simulink model "three_phase_dab"  (R2025b)
settings: Solver=ode23tb  StartTime=0.0  StopTime=simlength  FixedStep=tc  MaxStep=tc
values from neighbouring files (symbols this model uses):
  Idc_FS = max(Idab1_dc_nom,Idab2_dc_nom) * margin_factor    [init_model.m]
  tc = ts_dab/100    (= 4.16666666667e-07)    [init_model.m]
  Vdab2_dc_nom = 1500    [init_model.m]
  Vdc_FS = max(Vdab1_dc_nom,Vdab2_dc_nom) * margin_factor    [init_model.m]
libraries: fl_lib x19, nesl_utility x15, discrete_time_low_pass_filter x6, single_phase_transformer_lib x3, litium_ion_battery x2, pi_ctrl x2, three_phase_inverter_ideal_switch_based_model x2, three_phase_inverter_mosfet_based_with_thermal_model x2, three_phase_dab_modulator x1
settings Model: SimulationMode=accelerator  Creator=LTNBDA  LastModifiedBy=ltnbda
settings SolverCC: ZeroCrossControl=EnableAll  ZeroCrossAlgorithm=Adaptive  AlgebraicLoopSolver=TrustRegion  SolverResetMethod=Robust  AutoInsertRateTranBlk=on
settings DataIOCC: LimitDataPoints=on  MaxDataPoints=1  SaveFormat=Array  SignalLoggingSaveFormat=ModelDataLogs  SaveOutput=off  SignalLogging=off  DSMLogging=off  SaveTime=off  ReturnWorkspaceOutputs=off
settings OptimizationCC: ExpressionDepthLimit=2147483647.0  InitFltsAndDblsToZero=on  EfficientMapNaN2IntZero=off  LifeSpan=inf
settings DebuggingCC: SaveWithParameterizedLinksMsg=none  UnderspecifiedInitializationDetection=Classic  MergeDetectMultiDrivingBlocksExec=none  SignalResolutionControl=TryResolveAllWithWarning  SolverPrmCheckMsg=warning  MultiTaskDSMMsg=warning  MultiTaskCondExecSysMsg=none  MultiTaskRateTransMsg=warning  FcnCallInpInsideContextMsg=warning  StateNameClashWarn=warning  SFUnexpectedBacktrackingDiag=warning  SFNoUnconditionalDefaultTransitionDiag=warning  ArithmeticOperatorsInVariantConditions=warning
settings HardwareCC: ProdBitPerLong=64.0  ProdLargestAtomicFloat=None  ProdIntDivRoundTo=Undefined  ProdEndianess=Unspecified  ProdHWDeviceType=Generic->64-bit Embedded Processor (LP64)  TargetBitPerPointer=64.0  TargetBitPerSizeT=64.0  TargetBitPerPtrDiffT=64.0  TargetLongLongMode=on  TargetIntDivRoundTo=Zero  TargetEndianess=LittleEndian  TargetWordSize=64.0  TargetHWDeviceType=MATLAB Host  ProdEqTarget=off
settings ModelReferenceCC: EnableRefExpFcnMdlSchedulingChecks=on  PropagateSignalLabelsOutOfModel=off
settings SFSimCC: SimUseLocalCustomCode=off  CustomCodeUndefinedFunction=UseInterfaceOnly
settings RTWCC: RTWUseLocalCustomCode=off  GPUComputeCapability=3.5
settings CodeAppCC: MaxIdLength=128.0  StateflowObjectComments=on
settings GRTTargetCC: TargetLangStandard=C89/C90 (ANSI)  CombineOutputUpdateFcns=off  GRTInterface=on
settings ConfigComp: CovMetricSettings=dw  CovSaveCumulativeToWorkspaceVar=on  CovSaveSingleToWorkspaceVar=on  CovExternalEMLEnable=off
settings SimscapeCC: SimscapeNormalizeSystem=off

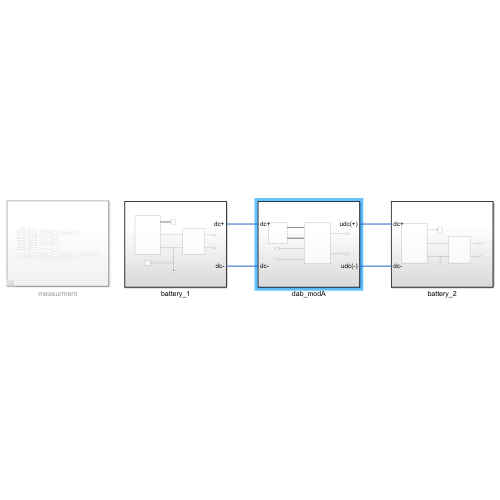
[thumbnail: Simulink's stored preview of the top-level diagram]
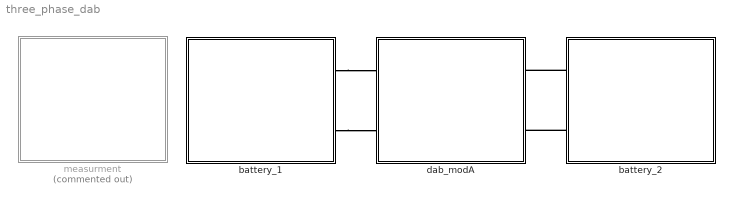
== system three_phase_dab ==
  battery_1 : Subsystem
  battery_2 : Subsystem
  dab_modA : Subsystem
  measurment : Subsystem  Commented=on
  connections:
  battery_2/RConn2 -- dab_modA/RConn2
  battery_2/RConn1 -- dab_modA/RConn1
  battery_1/RConn1 -- dab_modA/LConn1
  battery_1/RConn2 -- dab_modA/LConn2

== system three_phase_dab/battery_1 ==
  Electrical Reference1 : fl_lib/Electrical/Electrical Elements/Electrical Reference
  Solver Configuration : nesl_utility/Solver Configuration  PhysicalDomain=network_engine_domain  SubClassName=solver  LeftPortType=input  RightPortType=generic  Tones=[]  Harmonics=[]  SimulateNoise=off  Profile=off  UseLocalSampling=off  EnableSwitchedLinearOptims=on  FrequencyDomain=off  UseCCode=off  RelTol=0.001  AbsTol=0.001  MinStep=1e-09  ToWorkspace=off  RevertToSquareIcSolve=off  NumHomotopyIterations=100  PhasorMode=off  PhasorModeNumHarmonics=1  ConsistencySolver=NEWTON_FTOL  IndexReductionMethod=DerivativeReplacement  DoDC=off  ResidualTolerance=1e-09  ConsistencyTolSource=GLOBAL  ConsistencyAbsTol=0.001  ConsistencyRelTol=0.001  ConsistencyTolFactor=0.001  UseLocalSolver=on  LocalSolverChoice=NE_BACKWARD_EULER_ADVANCER  ResolveIndetEquations=on  FunctionEvalNumThread=1  LocalSolverSampleTime=tc  DoFixedCost=on  MaxNonlinIter=3  MaxModeIter=2  ComputeImpulses=off  ImpulseIterations=2  LinearAlgebra=auto  LinearAlgebraNumThread=0  EquationFormulation=NE_TIME_EF  DelaysMemoryBudget=1024  AutomaticFiltering=on  FilteringTimeConstant=0.001  PartitionStorageMethod=AS_NEEDED  PartitionMemoryBudget=1024  PartitionMethod=ROBUST  MultibodyUseLocalSolver=off  MultibodyLocalSolverChoice=ODE1  MultibodyLocalSolverSampleTime=0.001
  litium ion battery 1 : Scope
      settings: ActiveDisplayYMinimum=1095.5241232297076  ActiveDisplayYMaximum=1432.6160946881369  DataLoggingVariableName=ScopeData3
  litium_ion_battery : litium_ion_battery/litium_ion_battery  Q=50  number_of_cells=346  E_1=-1.031  E0=3.485  E1=0  E2=0  E3=0  Elog=-0.05  R0=0.035  R1=0.035  C1=0.5  M=125  alpha=35  soc_init=0.85  ts_battery=ts_battery  q1Kalman=q1Kalman  q2Kalman=q2Kalman  q3Kalman=q3Kalman  rKalman=rKalman  tc=tc
  single_phase_ui_measure : Subsystem
  dc+ : PMIOPort  Side=Right
  dc- : PMIOPort  Port=2  Side=Right
  wires:
  litium_ion_battery/1 -> litium ion battery 1/1
  connections:
  litium_ion_battery/RConn2 -- single_phase_ui_measure/LConn2 -- Electrical Reference1/LConn1 -- Solver Configuration/RConn1
  single_phase_ui_measure/RConn1 -- dc+/RConn1
  single_phase_ui_measure/LConn1 -- litium_ion_battery/RConn1
  dc-/RConn1 -- single_phase_ui_measure/RConn2

== system three_phase_dab/battery_2 ==
  Electrical Reference1 : fl_lib/Electrical/Electrical Elements/Electrical Reference
  litium ion battery 2 : Scope
      settings: ActiveDisplayYMinimum=-748.38980710578858  ActiveDisplayYMaximum=3166.4304287109808  DataLoggingVariableName=ScopeData3
  litium_ion_battery : litium_ion_battery/litium_ion_battery  Q=50  number_of_cells=346  E_1=-1.031  E0=3.485  E1=0  E2=0  E3=0  Elog=-0.05  R0=0.035  R1=0.035  C1=0.5  M=125  alpha=35  soc_init=0.85  ts_battery=ts_battery  q1Kalman=q1Kalman  q2Kalman=q2Kalman  q3Kalman=q3Kalman  rKalman=rKalman  tc=tc
  single_phase_ui_measure : Subsystem
  dc+ : PMIOPort  Side=Right
  dc- : PMIOPort  Port=2  Side=Right
  wires:
  litium_ion_battery/1 -> litium ion battery 2/1
  connections:
  dc-/RConn1 -- single_phase_ui_measure/RConn2
  single_phase_ui_measure/LConn1 -- litium_ion_battery/RConn1
  single_phase_ui_measure/RConn1 -- dc+/RConn1
  Electrical Reference1/LConn1 -- single_phase_ui_measure/LConn2 -- litium_ion_battery/RConn2

== system three_phase_dab/dab_modA ==
  dab_ctrl : Subsystem
  dcdc_with_galvanic_isolation : Subsystem
  udc(+) : PMIOPort  Side=Right
  udc(-) : PMIOPort  Port=2  Side=Right
  dc+ : PMIOPort  Port=3  Side=Left
  dc- : PMIOPort  Port=4  Side=Left
  wires:
  dab_ctrl/2(gate_commands_2) -> dcdc_with_galvanic_isolation/2(gate_commands_1)
  dab_ctrl/1(gate_commands_1) -> dcdc_with_galvanic_isolation/1(gate_commands_2)
  connections:
  udc(+)/RConn1 -- dcdc_with_galvanic_isolation/RConn1
  udc(-)/RConn1 -- dcdc_with_galvanic_isolation/RConn2
  dc-/RConn1 -- dcdc_with_galvanic_isolation/LConn2
  dc+/RConn1 -- dcdc_with_galvanic_isolation/LConn1

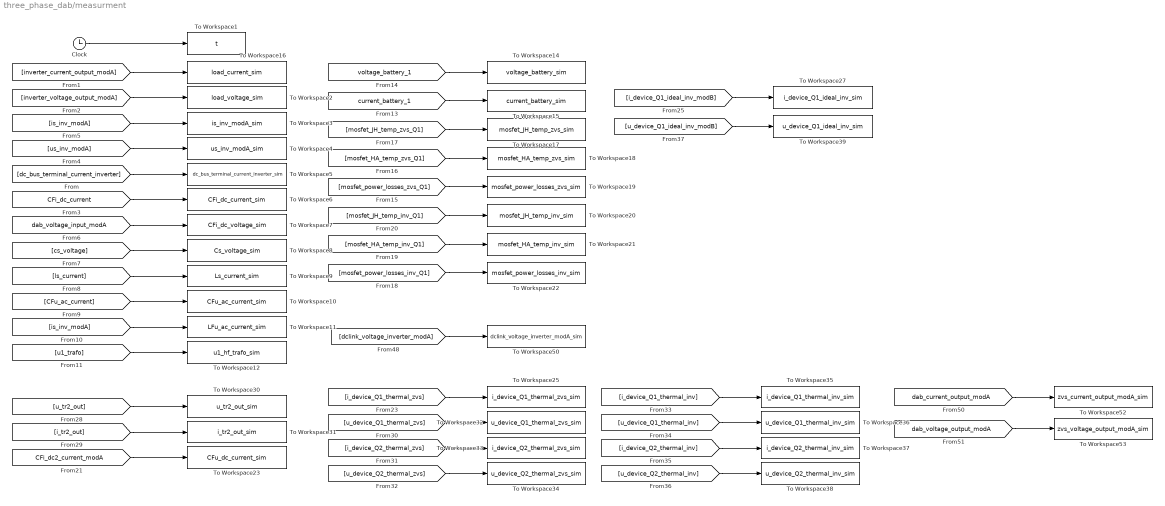
== system three_phase_dab/measurment ==
  Clock : Clock
  To Workspace1 : ToWorkspace  VariableName=t  SampleTime=tc
      settings: MaxDataPoints=Nc
  To Workspace10 : ToWorkspace  VariableName=CFu_ac_current_sim  SampleTime=tc
      settings: MaxDataPoints=Nc
  To Workspace11 : ToWorkspace  VariableName=LFu_ac_current_sim  SampleTime=tc
      settings: MaxDataPoints=Nc
  To Workspace12 : ToWorkspace  VariableName=u1_hf_trafo_sim  SampleTime=tc
      settings: MaxDataPoints=Nc
  To Workspace14 : ToWorkspace  VariableName=voltage_battery_sim  SampleTime=tc
      settings: MaxDataPoints=Nc
  To Workspace15 : ToWorkspace  VariableName=current_battery_sim  SampleTime=tc
      settings: MaxDataPoints=Nc
  To Workspace16 : ToWorkspace  VariableName=load_current_sim  SampleTime=tc
      settings: MaxDataPoints=Nc
  To Workspace17 : ToWorkspace  VariableName=mosfet_JH_temp_zvs_sim  SampleTime=tc
      settings: MaxDataPoints=Nc
  To Workspace18 : ToWorkspace  VariableName=mosfet_HA_temp_zvs_sim  SampleTime=tc
      settings: MaxDataPoints=Nc
  To Workspace19 : ToWorkspace  VariableName=mosfet_power_losses_zvs_sim  SampleTime=tc
      settings: MaxDataPoints=Nc
  To Workspace2 : ToWorkspace  VariableName=load_voltage_sim  SampleTime=tc
      settings: MaxDataPoints=Nc
  To Workspace20 : ToWorkspace  VariableName=mosfet_JH_temp_inv_sim  SampleTime=tc
      settings: MaxDataPoints=Nc
  To Workspace21 : ToWorkspace  VariableName=mosfet_HA_temp_inv_sim  SampleTime=tc
      settings: MaxDataPoints=Nc
  To Workspace22 : ToWorkspace  VariableName=mosfet_power_losses_inv_sim  SampleTime=tc
      settings: MaxDataPoints=Nc
  To Workspace23 : ToWorkspace  VariableName=CFu_dc_current_sim  SampleTime=tc
      settings: MaxDataPoints=Nc
  To Workspace25 : ToWorkspace  VariableName=i_device_Q1_thermal_zvs_sim  SampleTime=tc
      settings: MaxDataPoints=Nc
  To Workspace27 : ToWorkspace  VariableName=i_device_Q1_ideal_inv_sim  SampleTime=tc
      settings: MaxDataPoints=Nc
  To Workspace3 : ToWorkspace  VariableName=is_inv_modA_sim  SampleTime=tc
      settings: MaxDataPoints=Nc
  To Workspace30 : ToWorkspace  VariableName=u_tr2_out_sim  SampleTime=tc
      settings: MaxDataPoints=Nc
  To Workspace31 : ToWorkspace  VariableName=i_tr2_out_sim  SampleTime=tc
      settings: MaxDataPoints=Nc
  To Workspace32 : ToWorkspace  VariableName=u_device_Q1_thermal_zvs_sim  SampleTime=tc
      settings: MaxDataPoints=Nc
  To Workspace33 : ToWorkspace  VariableName=i_device_Q2_thermal_zvs_sim  SampleTime=tc
      settings: MaxDataPoints=Nc
  To Workspace34 : ToWorkspace  VariableName=u_device_Q2_thermal_zvs_sim  SampleTime=tc
      settings: MaxDataPoints=Nc
  To Workspace35 : ToWorkspace  VariableName=i_device_Q1_thermal_inv_sim  SampleTime=tc
      settings: MaxDataPoints=Nc
  To Workspace36 : ToWorkspace  VariableName=u_device_Q1_thermal_inv_sim  SampleTime=tc
      settings: MaxDataPoints=Nc
  To Workspace37 : ToWorkspace  VariableName=i_device_Q2_thermal_inv_sim  SampleTime=tc
      settings: MaxDataPoints=Nc
  To Workspace38 : ToWorkspace  VariableName=u_device_Q2_thermal_inv_sim  SampleTime=tc
      settings: MaxDataPoints=Nc
  To Workspace39 : ToWorkspace  VariableName=u_device_Q1_ideal_inv_sim  SampleTime=tc
      settings: MaxDataPoints=Nc
  To Workspace4 : ToWorkspace  VariableName=us_inv_modA_sim  SampleTime=tc
      settings: MaxDataPoints=Nc
  To Workspace5 : ToWorkspace  VariableName=dc_bus_terminal_current_inverter_sim  SampleTime=tc
      settings: MaxDataPoints=Nc
  To Workspace50 : ToWorkspace  VariableName=dclink_voltage_inverter_modA_sim  SampleTime=tc
      settings: MaxDataPoints=Nc
  To Workspace52 : ToWorkspace  VariableName=zvs_current_output_modA_sim  SampleTime=tc
      settings: MaxDataPoints=Nc
  To Workspace53 : ToWorkspace  VariableName=zvs_voltage_output_modA_sim  SampleTime=tc
      settings: MaxDataPoints=Nc
  To Workspace6 : ToWorkspace  VariableName=CFi_dc_current_sim  SampleTime=tc
      settings: MaxDataPoints=Nc
  To Workspace7 : ToWorkspace  VariableName=CFi_dc_voltage_sim  SampleTime=tc
      settings: MaxDataPoints=Nc
  To Workspace8 : ToWorkspace  VariableName=Cs_voltage_sim  SampleTime=tc
      settings: MaxDataPoints=Nc
  To Workspace9 : ToWorkspace  VariableName=Ls_current_sim  SampleTime=tc
      settings: MaxDataPoints=Nc
  wires:
  Clock/1 -> To Workspace1/1
  [inverter_current_output_modA] -> To Workspace16/1
  [inverter_voltage_output_modA] -> To Workspace2/1
  [is_inv_modA] -> To Workspace3/1
  [us_inv_modA] -> To Workspace4/1
  [dc_bus_terminal_current_inverter] -> To Workspace5/1
  [CFi_dc_current] -> To Workspace6/1
  [dab_voltage_input_modA] -> To Workspace7/1
  [cs_voltage] -> To Workspace8/1
  [ls_current] -> To Workspace9/1
  [CFu_ac_current] -> To Workspace10/1
  [is_inv_modA] -> To Workspace11/1
  [u1_trafo] -> To Workspace12/1
  [voltage_battery_1] -> To Workspace14/1
  [current_battery_1] -> To Workspace15/1
  [mosfet_JH_temp_zvs_Q1] -> To Workspace17/1
  [mosfet_HA_temp_zvs_Q1] -> To Workspace18/1
  [mosfet_power_losses_zvs_Q1] -> To Workspace19/1
  [mosfet_power_losses_inv_Q1] -> To Workspace22/1
  [mosfet_HA_temp_inv_Q1] -> To Workspace21/1
  [mosfet_JH_temp_inv_Q1] -> To Workspace20/1
  [CFi_dc2_current_modA] -> To Workspace23/1
  [i_device_Q1_thermal_zvs] -> To Workspace25/1
  [i_device_Q1_ideal_inv_modB] -> To Workspace27/1
  [u_tr2_out] -> To Workspace30/1
  [i_tr2_out] -> To Workspace31/1
  [u_device_Q1_thermal_zvs] -> To Workspace32/1
  [u_device_Q2_thermal_zvs] -> To Workspace34/1
  [i_device_Q2_thermal_zvs] -> To Workspace33/1
  [i_device_Q2_thermal_inv] -> To Workspace37/1
  [u_device_Q2_thermal_inv] -> To Workspace38/1
  [u_device_Q1_thermal_inv] -> To Workspace36/1
  [i_device_Q1_thermal_inv] -> To Workspace35/1
  [u_device_Q1_ideal_inv_modB] -> To Workspace39/1
  [dclink_voltage_inverter_modA] -> To Workspace50/1
  [dab_voltage_output_modA] -> To Workspace53/1
  [dab_current_output_modA] -> To Workspace52/1

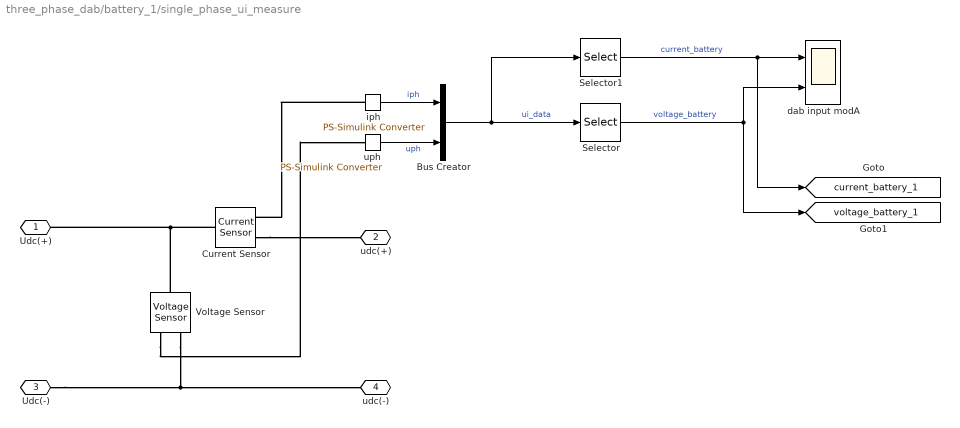
== system three_phase_dab/battery_1/single_phase_ui_measure ==
  Bus Creator : BusCreator  Inputs=2
  Current Sensor : fl_lib/Electrical/Electrical Sensors/Current Sensor
  Selector : Selector  InputPortWidth=2  IndexOptions=Index vector (dialog)  Indices=2  OutputSizes=1
  Selector1 : Selector  InputPortWidth=2  IndexOptions=Index vector (dialog)  Indices=1  OutputSizes=1
  Voltage Sensor : fl_lib/Electrical/Electrical Sensors/Voltage Sensor
  dab input modA : Scope  NumInputPorts=2
      settings: SampleTime=tc  ActiveDisplayYMinimum=-4428.9106738971032  ActiveDisplayYMaximum=4853.7975894934307  DataLoggingVariableName=ScopeData2
  iph : nesl_utility/PS-Simulink Converter  PhysicalDomain=network_engine_domain  SubClassName=ps_output  LeftPortType=input  RightPortType=output  PseudoPeriodic=off  Frequencies=[]  VectorFormat=1-D array  Unit=A  AffineConversion=off
  uph : nesl_utility/PS-Simulink Converter  PhysicalDomain=network_engine_domain  SubClassName=ps_output  LeftPortType=input  RightPortType=output  PseudoPeriodic=off  Frequencies=[]  VectorFormat=1-D array  Unit=V  AffineConversion=off
  Udc(+) : PMIOPort  Side=Left
  udc(+) : PMIOPort  Port=2  Side=Right
  Udc(-) : PMIOPort  Port=3  Side=Left
  udc(-) : PMIOPort  Port=4  Side=Right
  tag scope: current_battery_1=global, voltage_battery_1=global
  wires:
  Bus Creator/1 -> Selector/1, Selector1/1  "ui_data"
  iph/1 -> Bus Creator/1  "iph"
  uph/1 -> Bus Creator/2  "uph"
  Selector1/1 -> [current_battery_1], dab input modA/1  "current_battery"
  Selector/1 -> dab input modA/2, [voltage_battery_1]  "voltage_battery"
  connections:
  iph/LConn1 -- Current Sensor/RConn1
  Voltage Sensor/LConn1 -- Current Sensor/LConn1 -- Udc(+)/RConn1
  Current Sensor/RConn2 -- udc(+)/RConn1
  Voltage Sensor/RConn1 -- uph/LConn1
  Voltage Sensor/RConn2 -- Udc(-)/RConn1 -- udc(-)/RConn1

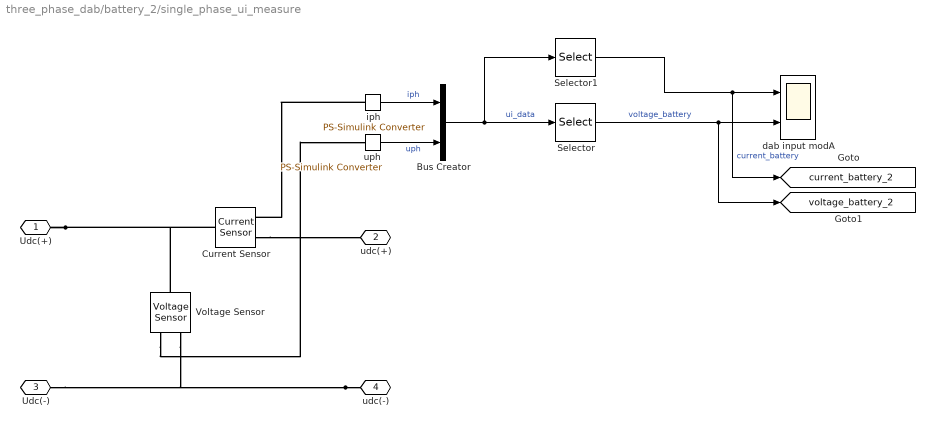
== system three_phase_dab/battery_2/single_phase_ui_measure ==
  Bus Creator : BusCreator  Inputs=2
  Current Sensor : fl_lib/Electrical/Electrical Sensors/Current Sensor
  Selector : Selector  InputPortWidth=2  IndexOptions=Index vector (dialog)  Indices=2  OutputSizes=1
  Selector1 : Selector  InputPortWidth=2  IndexOptions=Index vector (dialog)  Indices=1  OutputSizes=1
  Voltage Sensor : fl_lib/Electrical/Electrical Sensors/Voltage Sensor
  dab input modA : Scope  NumInputPorts=2
      settings: SampleTime=tc  ActiveDisplayYMinimum=-363.9315036867377  ActiveDisplayYMaximum=456.02820990604641  DataLoggingVariableName=ScopeData2
  iph : nesl_utility/PS-Simulink Converter  PhysicalDomain=network_engine_domain  SubClassName=ps_output  LeftPortType=input  RightPortType=output  PseudoPeriodic=off  Frequencies=[]  VectorFormat=1-D array  Unit=A  AffineConversion=off
  uph : nesl_utility/PS-Simulink Converter  PhysicalDomain=network_engine_domain  SubClassName=ps_output  LeftPortType=input  RightPortType=output  PseudoPeriodic=off  Frequencies=[]  VectorFormat=1-D array  Unit=V  AffineConversion=off
  Udc(+) : PMIOPort  Side=Left
  udc(+) : PMIOPort  Port=2  Side=Right
  Udc(-) : PMIOPort  Port=3  Side=Left
  udc(-) : PMIOPort  Port=4  Side=Right
  tag scope: current_battery_2=global, voltage_battery_2=global
  wires:
  Selector/1 -> [voltage_battery_2], dab input modA/2  "voltage_battery"
  Selector1/1 -> dab input modA/1, [current_battery_2]  "current_battery"
  uph/1 -> Bus Creator/2  "uph"
  iph/1 -> Bus Creator/1  "iph"
  Bus Creator/1 -> Selector1/1, Selector/1  "ui_data"
  connections:
  udc(-)/RConn1 -- Udc(-)/RConn1 -- Voltage Sensor/RConn2
  Voltage Sensor/RConn1 -- uph/LConn1
  Current Sensor/RConn2 -- udc(+)/RConn1
  Udc(+)/RConn1 -- Current Sensor/LConn1 -- Voltage Sensor/LConn1
  iph/LConn1 -- Current Sensor/RConn1

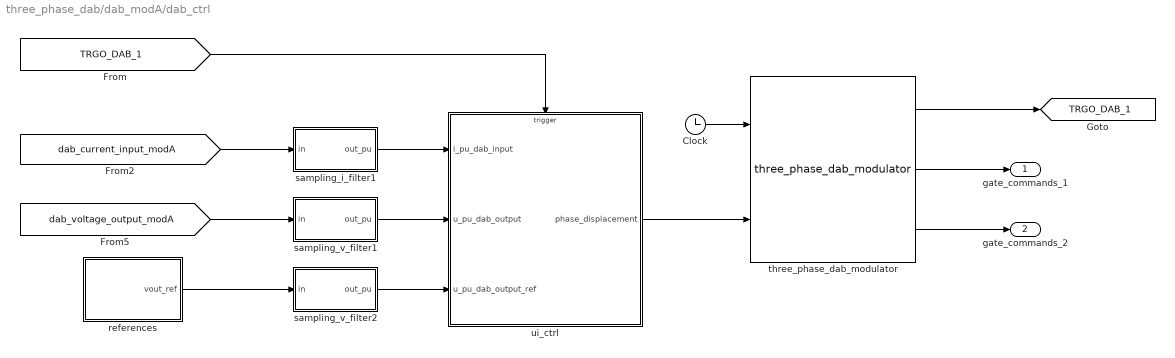
== system three_phase_dab/dab_modA/dab_ctrl ==
  Clock : Clock
  references : Subsystem
  sampling_i_filter1 : Subsystem
  sampling_v_filter1 : Subsystem
  sampling_v_filter2 : Subsystem
  three_phase_dab_modulator : three_phase_dab_modulator/three_phase_dab_modulator  fpwm=fPWM_DAB  tc=tc
  ui_ctrl : Subsystem
  gate_commands_1 : Outport
  gate_commands_2 : Outport  Port=2
  tag scope: TRGO_DAB_1=global
  wires:
  [dab_voltage_output_modA] -> sampling_v_filter1/1(in)
  [dab_current_input_modA] -> sampling_i_filter1/1(in)
  sampling_i_filter1/1(out_pu) -> ui_ctrl/1(i_pu_dab_input)
  sampling_v_filter1/1(out_pu) -> ui_ctrl/2(u_pu_dab_output)
  sampling_v_filter2/1(out_pu) -> ui_ctrl/3(u_pu_dab_output_ref)
  references/1(vout_ref) -> sampling_v_filter2/1(in)
  Clock/1 -> three_phase_dab_modulator/1
  three_phase_dab_modulator/1 -> [TRGO_DAB_1]
  [TRGO_DAB_1] -> ui_ctrl/Trigger
  ui_ctrl/1(phase_displacement) -> three_phase_dab_modulator/2
  three_phase_dab_modulator/2 -> gate_commands_1/1
  three_phase_dab_modulator/3 -> gate_commands_2/1

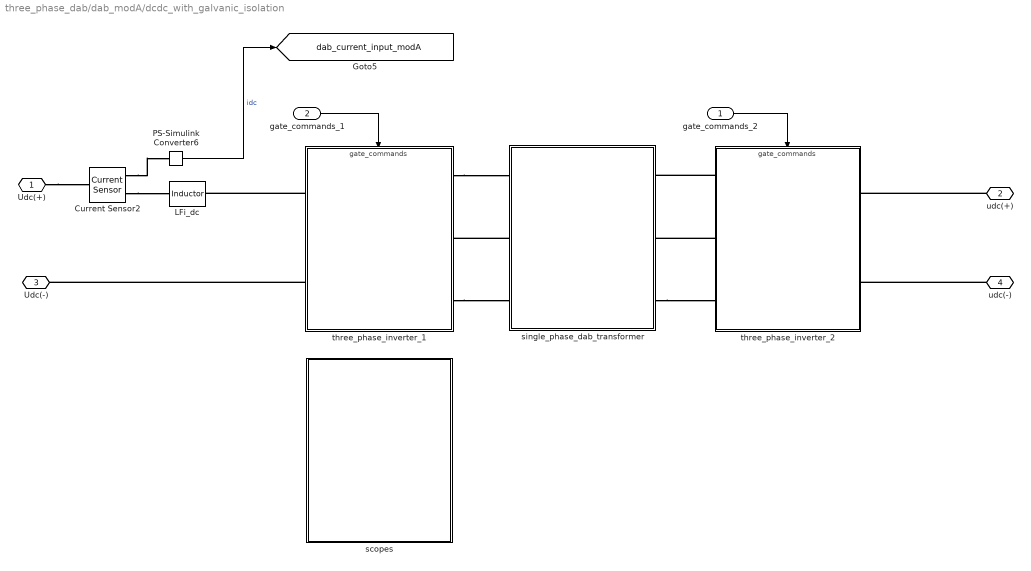
== system three_phase_dab/dab_modA/dcdc_with_galvanic_isolation ==
  gate_commands_2 : Inport
  gate_commands_1 : Inport  Port=2
  Current Sensor2 : fl_lib/Electrical/Electrical Sensors/Current Sensor
  LFi_dc : fl_lib/Electrical/Electrical Elements/Inductor  l=LFi_dc H  r=RLFi_dc Ohm  g=1e-9 1/Ohm  i_specify=off  i_priority=None  i=0 A  i_nominal_specify=off  i_nominal_value=1  i_nominal_unit=A  v_specify=off  v_priority=None  v=0 V  v_nominal_specify=off  v_nominal_value=1  v_nominal_unit=V  i_L_specify=off  i_L_priority=High  i_L=0 A  i_L_nominal_specify=off  i_L_nominal_value=1  i_L_nominal_unit=A
  PS-Simulink Converter6 : nesl_utility/PS-Simulink Converter  PhysicalDomain=network_engine_domain  SubClassName=ps_output  LeftPortType=input  RightPortType=output  PseudoPeriodic=off  Frequencies=[]  VectorFormat=1-D array  Unit=A  AffineConversion=on
  scopes : Subsystem
  single_phase_dab_transformer : Subsystem
  three_phase_inverter_1 : Subsystem
      settings: PortSchema="{\"entries\":[{\"content\":{\"sides\":[{\"content\":{\"connectorIds\":[\"LConn1\",\"LConn2\",\"LConn3\"]},\"type\":\"ConnectorPlacement.EquallySpacedRectSide\",\"uuid\":\"c872503a-61af-4937-bdf2-4de4f8645573\"},{\"content\":{\"connectorIds\":[\"RConn1\",\"RConn2\"],\"side\":\"RIGHT\"},\"type\":\"ConnectorPlacement.EquallySpacedRectSide\",\"uuid\":\"3b83f060-86a2-4569-84b5-d9f7c0485347\"},{\"content\":{\"connectorIds\":[\"In1\"],\"side\":\"TOP\"},\"type\":\"ConnectorPlacement.EquallySpacedRectSide\",\"uuid\":\"bf191d46-ce71-4d15-9dd0-24cc57253577\"}]},\"type\":\"ConnectorPlacement.EquallySpacedConnector\",\"uuid\":\"1b28ceee-25d0-45ae-a3c4-c2563f0d63ba\"}],\"packageUris\":[\"http://schema.mathworks.com/mf0/Connector/R2020b\"],\"version\":\"1.0\"}"
  three_phase_inverter_2 : Subsystem
      settings: PortSchema="{\"entries\":[{\"content\":{\"sides\":[{\"content\":{\"connectorIds\":[\"LConn1\",\"LConn2\",\"LConn3\"]},\"type\":\"ConnectorPlacement.EquallySpacedRectSide\",\"uuid\":\"c872503a-61af-4937-bdf2-4de4f8645573\"},{\"content\":{\"connectorIds\":[\"RConn1\",\"RConn2\"],\"side\":\"RIGHT\"},\"type\":\"ConnectorPlacement.EquallySpacedRectSide\",\"uuid\":\"3b83f060-86a2-4569-84b5-d9f7c0485347\"},{\"content\":{\"connectorIds\":[\"In1\"],\"side\":\"TOP\"},\"type\":\"ConnectorPlacement.EquallySpacedRectSide\",\"uuid\":\"bf191d46-ce71-4d15-9dd0-24cc57253577\"}]},\"type\":\"ConnectorPlacement.EquallySpacedConnector\",\"uuid\":\"1b28ceee-25d0-45ae-a3c4-c2563f0d63ba\"}],\"packageUris\":[\"http://schema.mathworks.com/mf0/Connector/R2020b\"],\"version\":\"1.0\"}"
  Udc(+) : PMIOPort  Side=Left
  udc(+) : PMIOPort  Port=2  Side=Right
  Udc(-) : PMIOPort  Port=3  Side=Left
  udc(-) : PMIOPort  Port=4  Side=Right
  tag scope: dab_current_input_modA=global
  wires:
  PS-Simulink Converter6/1 -> [dab_current_input_modA]  "idc"
  gate_commands_1/1 -> three_phase_inverter_1/1(gate_commands)
  gate_commands_2/1 -> three_phase_inverter_2/1(gate_commands)
  connections:
  single_phase_dab_transformer/LConn2 -- three_phase_inverter_1/LConn2
  three_phase_inverter_1/RConn1 -- LFi_dc/RConn1
  three_phase_inverter_1/RConn2 -- Udc(-)/RConn1
  three_phase_inverter_1/LConn1 -- single_phase_dab_transformer/LConn1
  udc(-)/RConn1 -- three_phase_inverter_2/RConn2
  Current Sensor2/RConn2 -- LFi_dc/LConn1
  Udc(+)/RConn1 -- Current Sensor2/LConn1
  Current Sensor2/RConn1 -- PS-Simulink Converter6/LConn1
  three_phase_inverter_2/LConn1 -- single_phase_dab_transformer/RConn1
  three_phase_inverter_2/LConn2 -- single_phase_dab_transformer/RConn2
  udc(+)/RConn1 -- three_phase_inverter_2/RConn1
  three_phase_inverter_1/LConn3 -- single_phase_dab_transformer/LConn3
  single_phase_dab_transformer/RConn3 -- three_phase_inverter_2/LConn3

== system three_phase_dab/dab_modA/dab_ctrl/references ==
  Rate Limiter : RateLimiter  RisingSlewLimit=Vdab2_dc_nom*10  FallingSlewLimit=-Vdab2_dc_nom*10  SampleTimeMode=inherited
  Vout_dc_nom : Step  Time=1e-3  After=Vdab2_dc_nom  SampleTime=0
  vout_ref : Outport
  wires:
  Rate Limiter/1 -> vout_ref/1
  Vout_dc_nom/1 -> Rate Limiter/1

== system three_phase_dab/dab_modA/dab_ctrl/sampling_i_filter1 ==
  in : Inport
  1/Ti3 : Gain  Gain=1/Idc_FS  OutDataTypeStr=double  SaturateOnIntegerOverflow=on  ParamDataTypeStr=Inherit: Same as input
  out_pu : Outport
  wires:
  in/1 -> 1/Ti3/1
  1/Ti3/1 -> out_pu/1

== system three_phase_dab/dab_modA/dab_ctrl/sampling_v_filter1 ==
  in : Inport
  1/Ti3 : Gain  Gain=1/Vdc_FS  OutDataTypeStr=double  SaturateOnIntegerOverflow=on  ParamDataTypeStr=Inherit: Same as input
  out_pu : Outport
  wires:
  in/1 -> 1/Ti3/1
  1/Ti3/1 -> out_pu/1

== system three_phase_dab/dab_modA/dab_ctrl/sampling_v_filter2 ==
  in : Inport
  1/Ti3 : Gain  Gain=1/Vdc_FS  OutDataTypeStr=double  SaturateOnIntegerOverflow=on  ParamDataTypeStr=Inherit: Same as input
  Saturation : Saturate  UpperLimit=1  LowerLimit=0  OutDataTypeStr=double
  out_pu : Outport
  wires:
  in/1 -> 1/Ti3/1
  1/Ti3/1 -> Saturation/1
  Saturation/1 -> out_pu/1

== system three_phase_dab/dab_modA/dab_ctrl/ui_ctrl ==
  i_pu_dab_input : Inport
  u_pu_dab_output : Inport  Port=2
  u_pu_dab_output_ref : Inport  Port=3
  Trigger : TriggerPort  VariantControl=(inherit)  PortDimensions=1
  dab_ctrl : Subsystem
  scopes : Subsystem
  phase_displacement : Outport
  wires:
  i_pu_dab_input/1 -> dab_ctrl/1(i_pu_dab_input)
  u_pu_dab_output/1 -> dab_ctrl/2(u_pu_dab_output)
  u_pu_dab_output_ref/1 -> dab_ctrl/3(u_pu_dab_output_ref)
  dab_ctrl/1(phase_displacement) -> phase_displacement/1

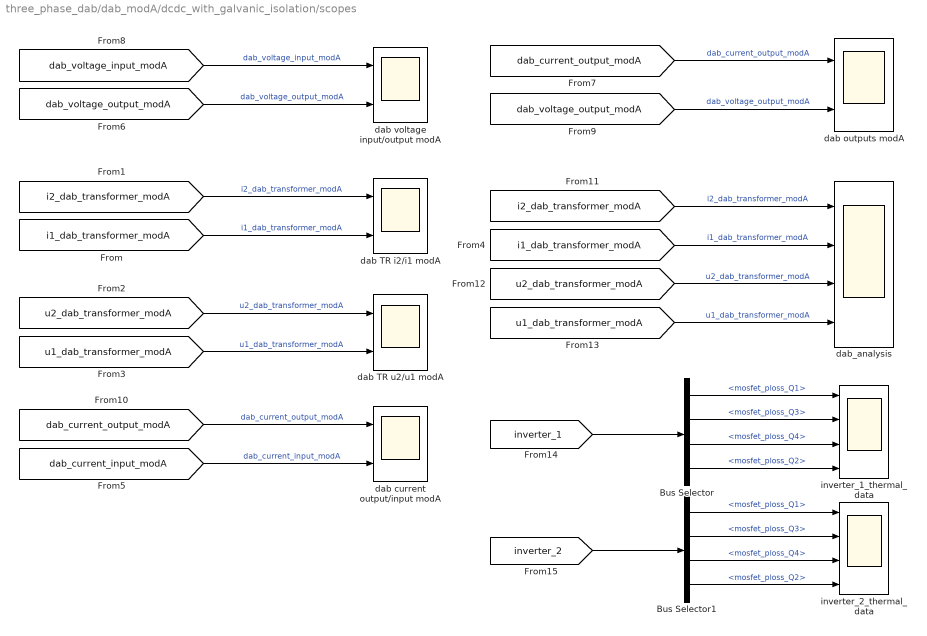
== system three_phase_dab/dab_modA/dcdc_with_galvanic_isolation/scopes ==
  Bus Selector : BusSelector  OutputSignals=mosfet_ploss_Q1,mosfet_ploss_Q3,mosfet_ploss_Q4,mosfet_ploss_Q2
  Bus Selector1 : BusSelector  OutputSignals=mosfet_ploss_Q1,mosfet_ploss_Q3,mosfet_ploss_Q4,mosfet_ploss_Q2
  dab TR i2/i1 modA : Scope  NumInputPorts=2
      settings: SampleTime=tc  ActiveDisplayYMinimum=-769.76570927697639  ActiveDisplayYMaximum=617.34679539784429  DataLoggingVariableName=ScopeData13
  dab TR u2/u1 modA : Scope  NumInputPorts=2
      settings: SampleTime=tc  ActiveDisplayYMinimum=-1578.7453878307324  ActiveDisplayYMaximum=1578.7340154658184  DataLoggingVariableName=ScopeData4
  dab current output/input modA : Scope  NumInputPorts=2
      settings: SampleTime=tc  ActiveDisplayYMinimum=-410.50779379600635  ActiveDisplayYMaximum=588.57119970360964  DataLoggingVariableName=ScopeData8
  dab outputs modA : Scope  NumInputPorts=2
      settings: SampleTime=tc  ActiveDisplayYMinimum=-911.87281827356537  ActiveDisplayYMaximum=678.26507696890121  DataLoggingVariableName=ScopeData6
  dab voltage input/output modA : Scope  NumInputPorts=2
      settings: SampleTime=tc  ActiveDisplayYMinimum=-158.19004113660858  ActiveDisplayYMaximum=1423.7103702331783  DataLoggingVariableName=ScopeData10
  dab_analysis : Scope  NumInputPorts=4
      settings: SampleTime=tc  ActiveDisplayYMinimum=-1875.7438152416184  ActiveDisplayYMaximum=1722.5640717808856  DataLoggingVariableName=ScopeData5
  inverter_1_thermal_data : Scope  NumInputPorts=4
      settings: SampleTime=tc  ActiveDisplayYMinimum=-410.50779379600635  ActiveDisplayYMaximum=588.57119970360964
  inverter_2_thermal_data : Scope  NumInputPorts=4
      settings: SampleTime=tc  ActiveDisplayYMinimum=-26.066888204230729  ActiveDisplayYMaximum=234.60199383807662  DataLoggingVariableName=ScopeData9
  wires:
  [dab_voltage_input_modA] -> dab voltage input/output modA/1  "dab_voltage_input_modA"
  [dab_current_output_modA] -> dab current output/input modA/1  "dab_current_output_modA"
  [dab_voltage_output_modA] -> dab voltage input/output modA/2  "dab_voltage_output_modA"
  [dab_current_input_modA] -> dab current output/input modA/2  "dab_current_input_modA"
  [i2_dab_transformer_modA] -> dab TR i2/i1 modA/1  "i2_dab_transformer_modA"
  [i1_dab_transformer_modA] -> dab TR i2/i1 modA/2  "i1_dab_transformer_modA"
  [u2_dab_transformer_modA] -> dab TR u2/u1 modA/1  "u2_dab_transformer_modA"
  [u1_dab_transformer_modA] -> dab TR u2/u1 modA/2  "u1_dab_transformer_modA"
  [dab_voltage_output_modA] -> dab outputs modA/2  "dab_voltage_output_modA"
  [dab_current_output_modA] -> dab outputs modA/1  "dab_current_output_modA"
  [i2_dab_transformer_modA] -> dab_analysis/1  "i2_dab_transformer_modA"
  [i1_dab_transformer_modA] -> dab_analysis/2  "i1_dab_transformer_modA"
  [u2_dab_transformer_modA] -> dab_analysis/3  "u2_dab_transformer_modA"
  [u1_dab_transformer_modA] -> dab_analysis/4  "u1_dab_transformer_modA"
  [inverter_1] -> Bus Selector/1
  Bus Selector/1 -> inverter_1_thermal_data/1  "<mosfet_ploss_Q1>"
  Bus Selector/2 -> inverter_1_thermal_data/2  "<mosfet_ploss_Q3>"
  Bus Selector/3 -> inverter_1_thermal_data/3  "<mosfet_ploss_Q4>"
  Bus Selector/4 -> inverter_1_thermal_data/4  "<mosfet_ploss_Q2>"
  Bus Selector1/4 -> inverter_2_thermal_data/4  "<mosfet_ploss_Q2>"
  Bus Selector1/3 -> inverter_2_thermal_data/3  "<mosfet_ploss_Q4>"
  Bus Selector1/2 -> inverter_2_thermal_data/2  "<mosfet_ploss_Q3>"
  Bus Selector1/1 -> inverter_2_thermal_data/1  "<mosfet_ploss_Q1>"
  [inverter_2] -> Bus Selector1/1

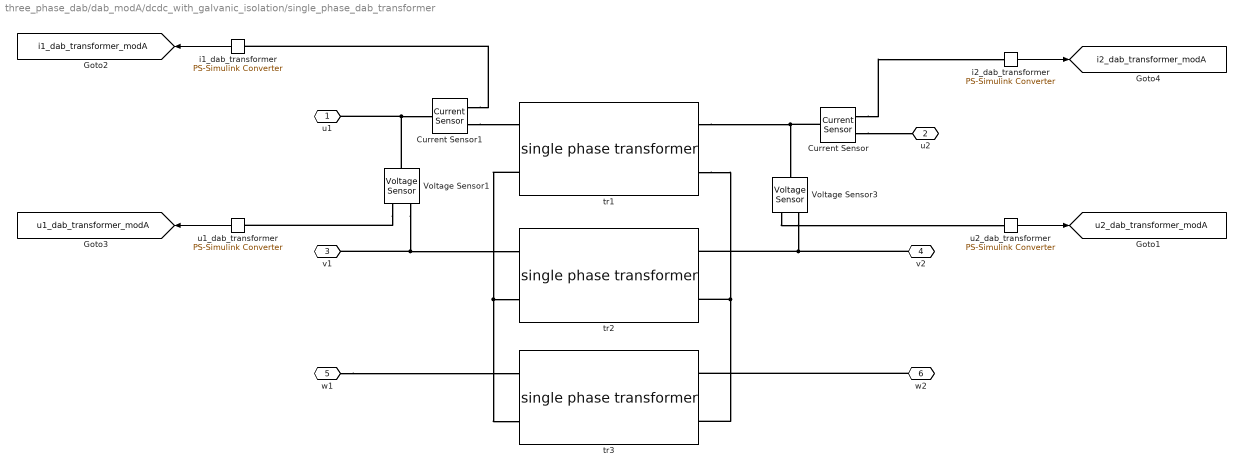
== system three_phase_dab/dab_modA/dcdc_with_galvanic_isolation/single_phase_dab_transformer ==
  Current Sensor : fl_lib/Electrical/Electrical Sensors/Current Sensor
  Current Sensor1 : fl_lib/Electrical/Electrical Sensors/Current Sensor
  Voltage Sensor1 : fl_lib/Electrical/Electrical Sensors/Voltage Sensor
  Voltage Sensor3 : fl_lib/Electrical/Electrical Sensors/Voltage Sensor
  i1_dab_transformer : nesl_utility/PS-Simulink Converter  PhysicalDomain=network_engine_domain  SubClassName=ps_output  LeftPortType=input  RightPortType=output  PseudoPeriodic=off  Frequencies=[]  VectorFormat=1-D array  Unit=A  AffineConversion=off
  i2_dab_transformer : nesl_utility/PS-Simulink Converter  PhysicalDomain=network_engine_domain  SubClassName=ps_output  LeftPortType=input  RightPortType=output  PseudoPeriodic=off  Frequencies=[]  VectorFormat=1-D array  Unit=A  AffineConversion=off
  tr1 : single_phase_transformer_lib/single phase transformer  Lm=lm_trafo H  n1=m1  n2=m2  Rd1=rd1_trafo Ohm  Rd2=rd2_trafo Ohm  Ld1=ld1_trafo H  Ld2=ld2_trafo H  Rfe=rfe_trafo Ohm  phi_specify=off  phi_priority=None  phi=0 V*s  phi_nominal_specify=off  phi_nominal_value=1  phi_nominal_unit=V*s  i1_specify=on  i1_priority=High  i1=0 A  i1_nominal_specify=off  i1_nominal_value=1  i1_nominal_unit=A  i2_specify=on  i2_priority=High  i2=0 A  i2_nominal_specify=off  i2_nominal_value=1  i2_nominal_unit=A  ife_specify=off  ife_priority=None  ife=0 A  ife_nominal_specify=off  ife_nominal_value=1  ife_nominal_unit=A  u1_specify=off  u1_priority=None  u1=0 V  u1_nominal_specify=off  u1_nominal_value=1  u1_nominal_unit=V  u2_specify=off  u2_priority=None  u2=0 V  u2_nominal_specify=off  u2_nominal_value=1  u2_nominal_unit=V
      settings: InternalSimscapePortConfiguration="{\"Bottom\":[],\"Left\":[{\"id\":\"u1_p\",\"label\":\"u1(+)\",\"type\":\"foundation.electrical.electrical\"},{\"id\":\"u1_n\",\"label\":\"u1(-)\",\"type\":\"foundation.electrical.electrical\"}],\"Right\":[{\"id\":\"u2_p\",\"label\":\"u2(+)\",\"type\":\"foundation.electrical.electrical\"},{\"id\":\"u2_n\",\"label\":\"u2(-)\",\"type\":\"foundation.electrical.electrical\"}],\"Top\":[]}"
  tr2 : single_phase_transformer_lib/single phase transformer  Lm=lm_trafo H  n1=m1  n2=m2  Rd1=rd1_trafo Ohm  Rd2=rd2_trafo Ohm  Ld1=ld1_trafo H  Ld2=ld2_trafo H  Rfe=rfe_trafo Ohm  phi_specify=off  phi_priority=None  phi=0 V*s  phi_nominal_specify=off  phi_nominal_value=1  phi_nominal_unit=V*s  i1_specify=on  i1_priority=High  i1=0 A  i1_nominal_specify=off  i1_nominal_value=1  i1_nominal_unit=A  i2_specify=on  i2_priority=High  i2=0 A  i2_nominal_specify=off  i2_nominal_value=1  i2_nominal_unit=A  ife_specify=off  ife_priority=None  ife=0 A  ife_nominal_specify=off  ife_nominal_value=1  ife_nominal_unit=A  u1_specify=off  u1_priority=None  u1=0 V  u1_nominal_specify=off  u1_nominal_value=1  u1_nominal_unit=V  u2_specify=off  u2_priority=None  u2=0 V  u2_nominal_specify=off  u2_nominal_value=1  u2_nominal_unit=V
      settings: InternalSimscapePortConfiguration="{\"Bottom\":[],\"Left\":[{\"id\":\"u1_p\",\"label\":\"u1(+)\",\"type\":\"foundation.electrical.electrical\"},{\"id\":\"u1_n\",\"label\":\"u1(-)\",\"type\":\"foundation.electrical.electrical\"}],\"Right\":[{\"id\":\"u2_p\",\"label\":\"u2(+)\",\"type\":\"foundation.electrical.electrical\"},{\"id\":\"u2_n\",\"label\":\"u2(-)\",\"type\":\"foundation.electrical.electrical\"}],\"Top\":[]}"
  tr3 : single_phase_transformer_lib/single phase transformer  Lm=lm_trafo H  n1=m1  n2=m2  Rd1=rd1_trafo Ohm  Rd2=rd2_trafo Ohm  Ld1=ld1_trafo H  Ld2=ld2_trafo H  Rfe=rfe_trafo Ohm  phi_specify=off  phi_priority=None  phi=0 V*s  phi_nominal_specify=off  phi_nominal_value=1  phi_nominal_unit=V*s  i1_specify=on  i1_priority=High  i1=0 A  i1_nominal_specify=off  i1_nominal_value=1  i1_nominal_unit=A  i2_specify=on  i2_priority=High  i2=0 A  i2_nominal_specify=off  i2_nominal_value=1  i2_nominal_unit=A  ife_specify=off  ife_priority=None  ife=0 A  ife_nominal_specify=off  ife_nominal_value=1  ife_nominal_unit=A  u1_specify=off  u1_priority=None  u1=0 V  u1_nominal_specify=off  u1_nominal_value=1  u1_nominal_unit=V  u2_specify=off  u2_priority=None  u2=0 V  u2_nominal_specify=off  u2_nominal_value=1  u2_nominal_unit=V
      settings: InternalSimscapePortConfiguration="{\"Bottom\":[],\"Left\":[{\"id\":\"u1_p\",\"label\":\"u1(+)\",\"type\":\"foundation.electrical.electrical\"},{\"id\":\"u1_n\",\"label\":\"u1(-)\",\"type\":\"foundation.electrical.electrical\"}],\"Right\":[{\"id\":\"u2_p\",\"label\":\"u2(+)\",\"type\":\"foundation.electrical.electrical\"},{\"id\":\"u2_n\",\"label\":\"u2(-)\",\"type\":\"foundation.electrical.electrical\"}],\"Top\":[]}"
  u1_dab_transformer : nesl_utility/PS-Simulink Converter  PhysicalDomain=network_engine_domain  SubClassName=ps_output  LeftPortType=input  RightPortType=output  PseudoPeriodic=off  Frequencies=[]  VectorFormat=1-D array  Unit=V  AffineConversion=on
  u2_dab_transformer : nesl_utility/PS-Simulink Converter  PhysicalDomain=network_engine_domain  SubClassName=ps_output  LeftPortType=input  RightPortType=output  PseudoPeriodic=off  Frequencies=[]  VectorFormat=1-D array  Unit=V  AffineConversion=on
  u1 : PMIOPort  Side=Left
  u2 : PMIOPort  Port=2  Side=Right
  v1 : PMIOPort  Port=3  Side=Left
  v2 : PMIOPort  Port=4  Side=Right
  w1 : PMIOPort  Port=5  Side=Left
  w2 : PMIOPort  Port=6  Side=Right
  tag scope: i1_dab_transformer_modA=global, i2_dab_transformer_modA=global, u1_dab_transformer_modA=global, u2_dab_transformer_modA=global
  wires:
  i2_dab_transformer/1 -> [i2_dab_transformer_modA]
  u2_dab_transformer/1 -> [u2_dab_transformer_modA]
  u1_dab_transformer/1 -> [u1_dab_transformer_modA]
  i1_dab_transformer/1 -> [i1_dab_transformer_modA]
  connections:
  Current Sensor/RConn1 -- i2_dab_transformer/LConn1
  Voltage Sensor3/RConn1 -- u2_dab_transformer/LConn1
  Voltage Sensor1/LConn1 -- u1/RConn1 -- Current Sensor1/LConn1
  Voltage Sensor1/RConn1 -- u1_dab_transformer/LConn1
  Current Sensor1/RConn1 -- i1_dab_transformer/LConn1
  Current Sensor/LConn1 -- tr1/RConn1 -- Voltage Sensor3/LConn1
  tr1/RConn2 -- tr2/RConn2 -- tr3/RConn2
  tr1/LConn2 -- tr2/LConn2 -- tr3/LConn2
  w1/RConn1 -- tr3/LConn1
  v2/RConn1 -- Voltage Sensor3/RConn2 -- tr2/RConn1
  w2/RConn1 -- tr3/RConn1
  Current Sensor1/RConn2 -- tr1/LConn1
  Voltage Sensor1/RConn2 -- v1/RConn1 -- tr2/LConn1
  Current Sensor/RConn2 -- u2/RConn1

== system three_phase_dab/dab_modA/dcdc_with_galvanic_isolation/three_phase_inverter_1 ==
  gate_commands : Inport
  dclink_1 : Subsystem
  three_phase_inverter_1 : Subsystem
  u : PMIOPort  Side=Left
  v : PMIOPort  Port=2  Side=Left
  Udc(+) : PMIOPort  Port=3  Side=Right
  Udc(-) : PMIOPort  Port=4  Side=Right
  w : PMIOPort  Port=5  Side=Left
  wires:
  gate_commands/1 -> three_phase_inverter_1/1(gate_commands)
  connections:
  Udc(+)/RConn1 -- dclink_1/LConn1
  Udc(-)/RConn1 -- dclink_1/LConn2
  dclink_1/RConn1 -- three_phase_inverter_1/LConn1
  three_phase_inverter_1/RConn1 -- u/RConn1
  three_phase_inverter_1/RConn2 -- v/RConn1
  three_phase_inverter_1/LConn2 -- dclink_1/RConn2
  w/RConn1 -- three_phase_inverter_1/RConn3

== system three_phase_dab/dab_modA/dcdc_with_galvanic_isolation/three_phase_inverter_2 ==
  gate_commands : Inport
  dclink_2 : Subsystem
  three_phase_inverter_2 : Subsystem
  u : PMIOPort  Side=Left
  v : PMIOPort  Port=2  Side=Left
  udc(+) : PMIOPort  Port=3  Side=Right
  udc(-) : PMIOPort  Port=4  Side=Right
  w : PMIOPort  Port=5  Side=Left
  wires:
  gate_commands/1 -> three_phase_inverter_2/1(gate_commands)
  connections:
  udc(+)/RConn1 -- dclink_2/RConn1
  udc(-)/RConn1 -- dclink_2/RConn2
  dclink_2/LConn1 -- three_phase_inverter_2/RConn1
  u/RConn1 -- three_phase_inverter_2/LConn1
  v/RConn1 -- three_phase_inverter_2/LConn2
  dclink_2/LConn2 -- three_phase_inverter_2/RConn2
  w/RConn1 -- three_phase_inverter_2/LConn3

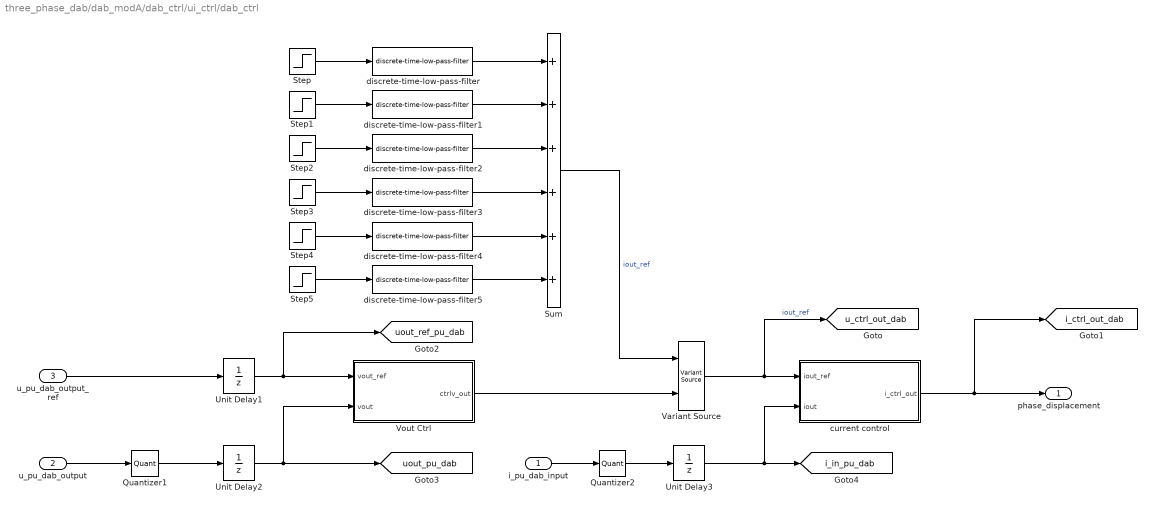
== system three_phase_dab/dab_modA/dab_ctrl/ui_ctrl/dab_ctrl ==
  i_pu_dab_input : Inport
  u_pu_dab_output : Inport  Port=2
  u_pu_dab_output_ref : Inport  Port=3
  Quantizer1 : Quantizer  QuantizationInterval=adc12_quantization
  Quantizer2 : Quantizer  QuantizationInterval=adc12_quantization
  Step : Step  Time=0.05  After=0.25
  Step1 : Step  Time=0.4  After=0.75
  Step2 : Step  Time=0.6  After=0.25
  Step3 : Step  Time=0.8  After=-1
  Step4 : Step  After=-0.75
  Step5 : Step  Time=1.25  After=-0.5
  Sum : Sum  Inputs=++++++
  Unit Delay1 : UnitDelay  SampleTime=-1  HasFrameUpgradeWarning=on
  Unit Delay2 : UnitDelay  SampleTime=-1  HasFrameUpgradeWarning=on
  Unit Delay3 : UnitDelay  SampleTime=-1  HasFrameUpgradeWarning=on
  Variant Source : VariantSource  VariantControls={true, false}
  Vout Ctrl : Subsystem
  current control : Subsystem
  discrete-time-low-pass-filter{,1..5} (6 alike) : discrete_time_low_pass_filter/discrete-time-low-pass-filter  tau=0.02  ts=ts_dab
  phase_displacement : Outport
  tag scope: i_ctrl_out_dab=global, i_in_pu_dab=global, u_ctrl_out_dab=global, uout_pu_dab=global, uout_ref_pu_dab=global
  wires:
  Vout Ctrl/1(ctrlv_out) -> Variant Source/2
  Variant Source/1 -> [u_ctrl_out_dab], current control/1(iout_ref)  "iout_ref"
  i_pu_dab_input/1 -> Quantizer2/1
  Sum/1 -> Variant Source/1  "iout_ref"
  current control/1(i_ctrl_out) -> phase_displacement/1, [i_ctrl_out_dab]
  Unit Delay3/1 -> current control/2(iout), [i_in_pu_dab]
  Unit Delay2/1 -> [uout_pu_dab], Vout Ctrl/2(vout)
  Unit Delay1/1 -> Vout Ctrl/1(vout_ref), [uout_ref_pu_dab]
  u_pu_dab_output/1 -> Quantizer1/1
  Step/1 -> discrete-time-low-pass-filter/1
  Step1/1 -> discrete-time-low-pass-filter1/1
  Step2/1 -> discrete-time-low-pass-filter2/1
  Step3/1 -> discrete-time-low-pass-filter3/1
  Step4/1 -> discrete-time-low-pass-filter4/1
  Step5/1 -> discrete-time-low-pass-filter5/1
  discrete-time-low-pass-filter/1 -> Sum/1
  discrete-time-low-pass-filter1/1 -> Sum/2
  discrete-time-low-pass-filter2/1 -> Sum/3
  discrete-time-low-pass-filter3/1 -> Sum/4
  discrete-time-low-pass-filter4/1 -> Sum/5
  discrete-time-low-pass-filter5/1 -> Sum/6
  u_pu_dab_output_ref/1 -> Unit Delay1/1
  Quantizer1/1 -> Unit Delay2/1
  Quantizer2/1 -> Unit Delay3/1

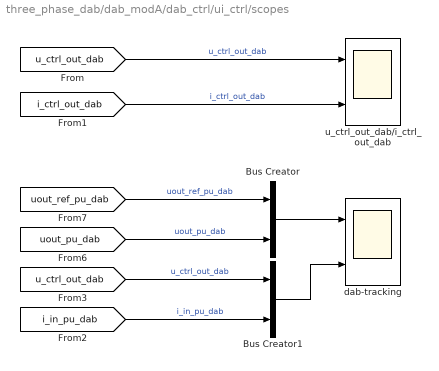
== system three_phase_dab/dab_modA/dab_ctrl/ui_ctrl/scopes ==
  Bus Creator : BusCreator  Inputs=2
  Bus Creator1 : BusCreator  Inputs=2
  dab-tracking : Scope  NumInputPorts=2
      settings: ActiveDisplayYMinimum=-2.3268130293516371  ActiveDisplayYMaximum=3.0115670177424061  DataLoggingVariableName=ScopeData7
  u_ctrl_out_dab/i_ctrl_out_dab : Scope  NumInputPorts=2
      settings: ActiveDisplayYMinimum=-1.2812486231311795  ActiveDisplayYMaximum=1.531237608180616
  wires:
  Bus Creator1/1 -> dab-tracking/2
  Bus Creator/1 -> dab-tracking/1
  [i_ctrl_out_dab] -> u_ctrl_out_dab/i_ctrl_out_dab/2  "i_ctrl_out_dab"
  [i_in_pu_dab] -> Bus Creator1/2  "i_in_pu_dab"
  [uout_ref_pu_dab] -> Bus Creator/1  "uout_ref_pu_dab"
  [u_ctrl_out_dab] -> u_ctrl_out_dab/i_ctrl_out_dab/1  "u_ctrl_out_dab"
  [u_ctrl_out_dab] -> Bus Creator1/1  "u_ctrl_out_dab"
  [uout_pu_dab] -> Bus Creator/2  "uout_pu_dab"

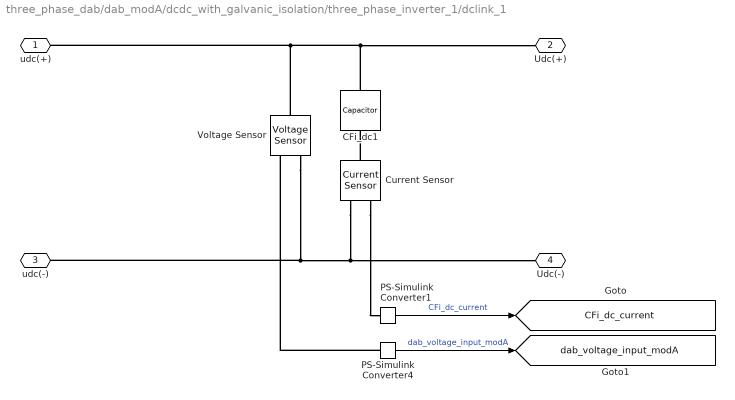
== system three_phase_dab/dab_modA/dcdc_with_galvanic_isolation/three_phase_inverter_1/dclink_1 ==
  CFi_dc1 : fl_lib/Electrical/Electrical Elements/Capacitor  c=CFi_dc1 F  r=RCFi_dc1_internal Ohm  g=0 1/Ohm  i_specify=off  i_priority=None  i=0 A  i_nominal_specify=off  i_nominal_value=1  i_nominal_unit=A  v_specify=off  v_priority=None  v=0 V  v_nominal_specify=off  v_nominal_value=1  v_nominal_unit=V  vc_specify=off  vc_priority=High  vc=0 V  vc_nominal_specify=off  vc_nominal_value=1  vc_nominal_unit=V
  Current Sensor : fl_lib/Electrical/Electrical Sensors/Current Sensor
  PS-Simulink Converter1 : nesl_utility/PS-Simulink Converter  PhysicalDomain=network_engine_domain  SubClassName=ps_output  LeftPortType=input  RightPortType=output  PseudoPeriodic=off  Frequencies=[]  VectorFormat=1-D array  Unit=A  AffineConversion=on
  PS-Simulink Converter4 : nesl_utility/PS-Simulink Converter  PhysicalDomain=network_engine_domain  SubClassName=ps_output  LeftPortType=input  RightPortType=output  PseudoPeriodic=off  Frequencies=[]  VectorFormat=1-D array  Unit=V  AffineConversion=on
  Voltage Sensor : fl_lib/Electrical/Electrical Sensors/Voltage Sensor
  udc(+) : PMIOPort  Side=Left
  Udc(+) : PMIOPort  Port=2  Side=Right
  udc(-) : PMIOPort  Port=3  Side=Left
  Udc(-) : PMIOPort  Port=4  Side=Right
  tag scope: CFi_dc_current=global, dab_voltage_input_modA=global
  wires:
  PS-Simulink Converter4/1 -> [dab_voltage_input_modA]  "dab_voltage_input_modA"
  PS-Simulink Converter1/1 -> [CFi_dc_current]  "CFi_dc_current"
  connections:
  Current Sensor/RConn1 -- PS-Simulink Converter1/LConn1
  PS-Simulink Converter4/LConn1 -- Voltage Sensor/RConn1
  Current Sensor/LConn1 -- CFi_dc1/RConn1
  Voltage Sensor/RConn2 -- Current Sensor/RConn2 -- Udc(-)/RConn1 -- udc(-)/RConn1
  CFi_dc1/LConn1 -- Udc(+)/RConn1 -- udc(+)/RConn1 -- Voltage Sensor/LConn1

== system three_phase_dab/dab_modA/dcdc_with_galvanic_isolation/three_phase_inverter_1/three_phase_inverter_1 ==
  gate_commands : Inport
  three_phase_inverter_ideal_switch_based_model : three_phase_inverter_ideal_switch_based_model/three phase inverter ideal switch based model  Commented=on  Ron_ideal_switch=Rds_on  Vth=Vth  Vgamma=Vdon_diode  Rdon_diode=Rdon_diode  Csnubber=Csnubber  Rsnubber=Rsnubber
  three_phase_inverter_mosfet_based_with_thermal_model : three_phase_inverter_mosfet_based_with_thermal_model/three phase inverter mosfet based with thermal model  mass_heatsink=0.2  specific_heat=cp_al  rth_mosfet_HA=Rth_mosfet_HA  rth_mosfet_JH=Rth_mosfet_JH  Rds_on=Rds_on  Vth=Vth  Eon=Eon  Eoff=Eoff  Voff_sw_loss=Voff_sw_losses  Ion_sw_loss=Ion_sw_losses  Vdon_diode=Vdon_diode  Rdon_diode=Rdon_diode  JunctionTermalMass=JunctionTermalMass  Tambient=Tambient  DThs_init=DThs_init
  udc(+) : PMIOPort  Side=Left
  u : PMIOPort  Port=2  Side=Right
  v : PMIOPort  Port=3  Side=Right
  udc(-) : PMIOPort  Port=4  Side=Left
  w : PMIOPort  Port=5  Side=Right
  tag scope: inverter_1=global
  wires:
  gate_commands/1 -> three_phase_inverter_ideal_switch_based_model/1, three_phase_inverter_mosfet_based_with_thermal_model/1
  three_phase_inverter_mosfet_based_with_thermal_model/1 -> [inverter_1]
  connections:
  u/RConn1 -- three_phase_inverter_ideal_switch_based_model/RConn1 -- three_phase_inverter_mosfet_based_with_thermal_model/RConn1
  v/RConn1 -- three_phase_inverter_ideal_switch_based_model/RConn2 -- three_phase_inverter_mosfet_based_with_thermal_model/RConn2
  udc(-)/RConn1 -- three_phase_inverter_ideal_switch_based_model/LConn2 -- three_phase_inverter_mosfet_based_with_thermal_model/LConn2
  w/RConn1 -- three_phase_inverter_ideal_switch_based_model/RConn3 -- three_phase_inverter_mosfet_based_with_thermal_model/RConn3
  udc(+)/RConn1 -- three_phase_inverter_ideal_switch_based_model/LConn1 -- three_phase_inverter_mosfet_based_with_thermal_model/LConn1

== system three_phase_dab/dab_modA/dcdc_with_galvanic_isolation/three_phase_inverter_2/dclink_2 ==
  CFi_dc2 : fl_lib/Electrical/Electrical Elements/Capacitor  c=CFi_dc2 F  r=RCFi_dc2_internal Ohm  g=0 1/Ohm  i_specify=off  i_priority=None  i=0 A  i_nominal_specify=off  i_nominal_value=1  i_nominal_unit=A  v_specify=off  v_priority=None  v=0 V  v_nominal_specify=off  v_nominal_value=1  v_nominal_unit=V  vc_specify=off  vc_priority=High  vc=0 V  vc_nominal_specify=off  vc_nominal_value=1  vc_nominal_unit=V
  Current Sensor2 : fl_lib/Electrical/Electrical Sensors/Current Sensor
  PS-Simulink Converter6 : nesl_utility/PS-Simulink Converter  PhysicalDomain=network_engine_domain  SubClassName=ps_output  LeftPortType=input  RightPortType=output  PseudoPeriodic=off  Frequencies=[]  VectorFormat=1-D array  Unit=A  AffineConversion=on
  ui_measure : Subsystem
  Udc(+) : PMIOPort  Side=Left
  Udc(-) : PMIOPort  Port=2  Side=Left
  udc(+) : PMIOPort  Port=3  Side=Right
  udc(-) : PMIOPort  Port=4  Side=Right
  tag scope: CFi_dc2_current_modA=global
  wires:
  PS-Simulink Converter6/1 -> [CFi_dc2_current_modA]  "CFi_dc2_current_modA"
  connections:
  CFi_dc2/RConn1 -- Current Sensor2/LConn1
  PS-Simulink Converter6/LConn1 -- Current Sensor2/RConn1
  Current Sensor2/RConn2 -- Udc(-)/RConn1 -- ui_measure/RConn2
  CFi_dc2/LConn1 -- ui_measure/RConn1 -- Udc(+)/RConn1
  ui_measure/LConn2 -- udc(-)/RConn1
  ui_measure/LConn1 -- udc(+)/RConn1

== system three_phase_dab/dab_modA/dcdc_with_galvanic_isolation/three_phase_inverter_2/three_phase_inverter_2 ==
  gate_commands : Inport
  three_phase_inverter_ideal_switch_based_model : three_phase_inverter_ideal_switch_based_model/three phase inverter ideal switch based model  Commented=on  Ron_ideal_switch=Rds_on  Vth=Vth  Vgamma=Vdon_diode  Rdon_diode=Rdon_diode  Csnubber=Csnubber  Rsnubber=Rsnubber
      link override ideal_switch_3: SourceBlock=three_phase_inverter_ideal_switch_based_model/three_phase_inverter_ideal_switch_based_model/ideal_switch_1
  three_phase_inverter_mosfet_based_with_thermal_model : three_phase_inverter_mosfet_based_with_thermal_model/three phase inverter mosfet based with thermal model  mass_heatsink=0.2  specific_heat=cp_al  rth_mosfet_HA=Rth_mosfet_HA  rth_mosfet_JH=Rth_mosfet_JH  Rds_on=Rds_on  Vth=Vth  Eon=Eon  Eoff=Eoff  Voff_sw_loss=Voff_sw_losses  Ion_sw_loss=Ion_sw_losses  Vdon_diode=Vdon_diode  Rdon_diode=Rdon_diode  JunctionTermalMass=JunctionTermalMass  Tambient=Tambient  DThs_init=DThs_init
  udc(+) : PMIOPort  Side=Right
  u : PMIOPort  Port=2  Side=Left
  v : PMIOPort  Port=3  Side=Left
  udc(-) : PMIOPort  Port=4  Side=Right
  w : PMIOPort  Port=5  Side=Left
  tag scope: inverter_2=global
  wires:
  gate_commands/1 -> three_phase_inverter_ideal_switch_based_model/1, three_phase_inverter_mosfet_based_with_thermal_model/1
  three_phase_inverter_mosfet_based_with_thermal_model/1 -> [inverter_2]
  connections:
  three_phase_inverter_mosfet_based_with_thermal_model/LConn2 -- three_phase_inverter_ideal_switch_based_model/LConn2 -- udc(-)/RConn1
  three_phase_inverter_mosfet_based_with_thermal_model/LConn1 -- udc(+)/RConn1 -- three_phase_inverter_ideal_switch_based_model/LConn1
  three_phase_inverter_mosfet_based_with_thermal_model/RConn1 -- u/RConn1 -- three_phase_inverter_ideal_switch_based_model/RConn1
  three_phase_inverter_mosfet_based_with_thermal_model/RConn3 -- w/RConn1 -- three_phase_inverter_ideal_switch_based_model/RConn3
  three_phase_inverter_mosfet_based_with_thermal_model/RConn2 -- v/RConn1 -- three_phase_inverter_ideal_switch_based_model/RConn2

== system three_phase_dab/dab_modA/dab_ctrl/ui_ctrl/dab_ctrl/Vout Ctrl ==
  vout_ref : Inport
  vout : Inport  Port=2
  pi_ctrl : pi_ctrl/pi_ctrl  kp=kp_v_dab  ki=ki_v_dab  ts=ts_dab  lim_up=2  lim_down=-2
  ctrlv_out : Outport
  wires:
  vout_ref/1 -> pi_ctrl/1
  vout/1 -> pi_ctrl/2
  pi_ctrl/1 -> ctrlv_out/1

== system three_phase_dab/dab_modA/dab_ctrl/ui_ctrl/dab_ctrl/current control ==
  iout_ref : Inport
  iout : Inport  Port=2
  Gain : Gain
  Gain1 : Gain  Gain=-1
  i_out_dab_tracking : Scope  NumInputPorts=3
      settings: ActiveDisplayYMinimum=-3.68017578125  ActiveDisplayYMaximum=5.81201171875  DataLoggingVariableName=ScopeData12
  pi_ctrl : pi_ctrl/pi_ctrl  kp=kp_i_dab  ki=ki_i_dab  ts=ts_dab  lim_up=1  lim_down=-1
  i_ctrl_out : Outport
  wires:
  iout_ref/1 -> pi_ctrl/1, i_out_dab_tracking/1, Gain/1  "i_out_dab_ref"
  iout/1 -> pi_ctrl/2, i_out_dab_tracking/2  "i_out_dab"
  Gain/1 -> pi_ctrl/3
  pi_ctrl/1 -> Gain1/1
  Gain1/1 -> i_out_dab_tracking/3, i_ctrl_out/1  "i_ctrl_out"

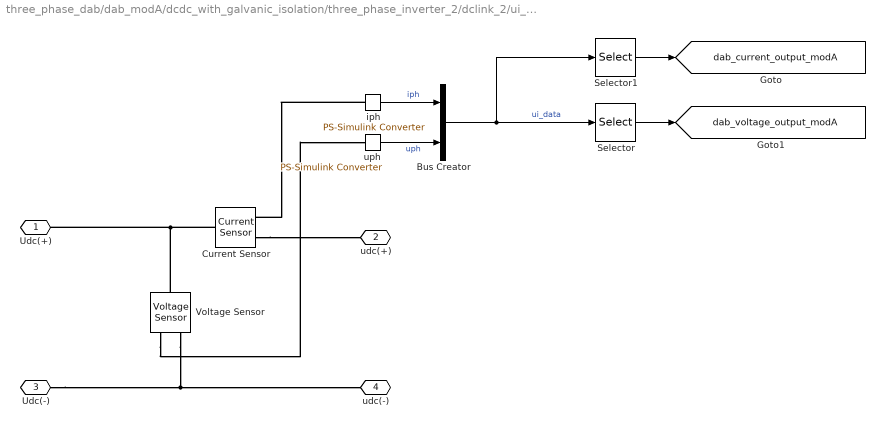
== system three_phase_dab/dab_modA/dcdc_with_galvanic_isolation/three_phase_inverter_2/dclink_2/ui_measure ==
  Bus Creator : BusCreator  Inputs=2
  Current Sensor : fl_lib/Electrical/Electrical Sensors/Current Sensor
  Selector : Selector  InputPortWidth=2  IndexOptions=Index vector (dialog)  Indices=2  OutputSizes=1
  Selector1 : Selector  InputPortWidth=2  IndexOptions=Index vector (dialog)  Indices=1  OutputSizes=1
  Voltage Sensor : fl_lib/Electrical/Electrical Sensors/Voltage Sensor
  iph : nesl_utility/PS-Simulink Converter  PhysicalDomain=network_engine_domain  SubClassName=ps_output  LeftPortType=input  RightPortType=output  PseudoPeriodic=off  Frequencies=[]  VectorFormat=1-D array  Unit=A  AffineConversion=off
  uph : nesl_utility/PS-Simulink Converter  PhysicalDomain=network_engine_domain  SubClassName=ps_output  LeftPortType=input  RightPortType=output  PseudoPeriodic=off  Frequencies=[]  VectorFormat=1-D array  Unit=V  AffineConversion=off
  Udc(+) : PMIOPort  Side=Left
  udc(+) : PMIOPort  Port=2  Side=Right
  Udc(-) : PMIOPort  Port=3  Side=Left
  udc(-) : PMIOPort  Port=4  Side=Right
  tag scope: dab_current_output_modA=global, dab_voltage_output_modA=global
  wires:
  Selector1/1 -> [dab_current_output_modA]
  Selector/1 -> [dab_voltage_output_modA]
  Bus Creator/1 -> Selector/1, Selector1/1  "ui_data"
  iph/1 -> Bus Creator/1  "iph"
  uph/1 -> Bus Creator/2  "uph"
  connections:
  iph/LConn1 -- Current Sensor/RConn1
  Voltage Sensor/LConn1 -- Current Sensor/LConn1 -- Udc(+)/RConn1
  Current Sensor/RConn2 -- udc(+)/RConn1
  Voltage Sensor/RConn1 -- uph/LConn1
  Voltage Sensor/RConn2 -- Udc(-)/RConn1 -- udc(-)/RConn1
